simulink model "myModel2"  (R2018b)
settings: Solver=VariableStepAuto  StartTime=0.0  StopTime=3  RelTol=1e-3
settings Model: Creator=lorenzo  LastModifiedBy=lorenzo

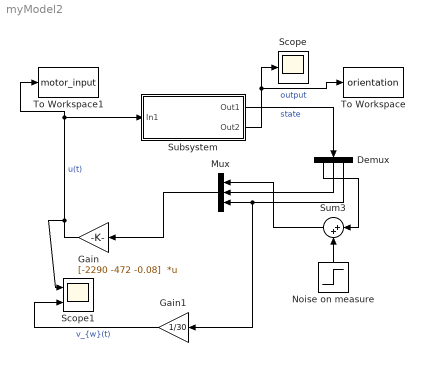
== system myModel2 ==
  Demux : Demux  Outputs=3
  Gain : Gain  Gain=[-2290 -472 -0.08]  Multiplication=Matrix(K*u) (u vector)
  Gain1 : Gain  Gain=1/30
  Mux : Mux  Inputs=3
  "Noise on measure " : Step  Time=1.5  After=0.2/107.47  SampleTime=0
  Scope : Scope
  Scope1 : Scope  NumInputPorts=2
  Subsystem : Subsystem
  Sum3 : Sum  Inputs=|++
  To Workspace : ToWorkspace  VariableName=orientation  SaveFormat=Timeseries  SampleTime=-1
  To Workspace1 : ToWorkspace  VariableName=motor_input  SaveFormat=Timeseries  SampleTime=-1
  wires:
  Demux/3 -> Gain1/1, Mux/3
  Demux/2 -> Mux/2
  Gain/1 -> Scope1/1, To Workspace1/1, Subsystem/1(In1)  "u(t)"
  Subsystem/2(Out2) -> To Workspace/1, Scope/1  "output"
  Subsystem/1(Out1) -> Demux/1  "state"
  "Noise on measure "/1 -> Sum3/2
  Mux/1 -> Gain/1
  Demux/1 -> Sum3/1
  Sum3/1 -> Mux/1
  Gain1/1 -> Scope1/2  "v_{w}(t)"

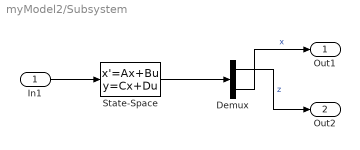
== system myModel2/Subsystem ==
  In1 : Inport
  Demux : Demux  Outputs=2
  State-Space : StateSpace  A=[0 1 0; 23.5031 0 0.0045; -23.5031 0 -19.9513]  B=[0; 0.1393; -621.6819]  C=[107.47 0 0; 1 0 0; 0 1 0; 0 0 1]  D=[0; 0; 0; 0]  InitialCondition=[0.2/107.47;0;0]
  Out1 : Outport
  Out2 : Outport  Port=2
  wires:
  State-Space/1 -> Demux/1
  In1/1 -> State-Space/1
  Demux/1 -> Out2/1  "z"
  Demux/2 -> Out1/1  "x"
